simulink model "momentum_unload_test_super_simple"  (R2016b)
settings: Solver=VariableStepAuto  StartTime=0.0  StopTime=10  RelTol=1e-3
libraries: dynamics_lib x1, environment_lib x1, momentum_dump_lib x1, actuators_lib x1
settings Model: Creator=taylorreynolds  LastModifiedBy=evich

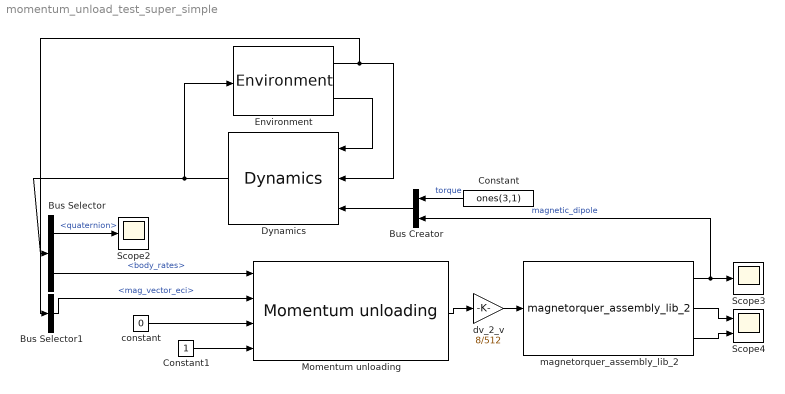
== system momentum_unload_test_super_simple ==
  Bus Creator : BusCreator  Inputs=2
  Bus Selector : BusSelector  OutputSignals=quaternion,body_rates
  Bus Selector1 : BusSelector  OutputSignals=mag_vector_eci
  Constant : Constant  Value=ones(3,1)
  Constant1 : Constant
  Dynamics : dynamics_lib/Dynamics
  Environment : environment_lib/Environment
  Momentum unloading : momentum_dump_lib/Momentum unloading
  Scope2 : Scope
  Scope3 : Scope
  Scope4 : Scope  NumInputPorts=2
  constant : Constant  Value=0
  dv_2_v : Gain  Gain=8/512
  magnetorquer_assembly_lib_2 : actuators_lib/Actuators/magnetorquer_assembly_lib_2
  wires:
  Environment/1 -> Bus Selector1/1, Dynamics/2
  Dynamics/1 -> Environment/1, Bus Selector/1
  Bus Selector/2 -> Momentum unloading/1  "<body_rates>"
  Bus Selector/1 -> Scope2/1  "<quaternion>"
  Bus Creator/1 -> Dynamics/3
  magnetorquer_assembly_lib_2/1 -> Scope3/1, Bus Creator/2  "magnetic_dipole"
  constant/1 -> Momentum unloading/3
  Momentum unloading/1 -> dv_2_v/1
  dv_2_v/1 -> magnetorquer_assembly_lib_2/1
  magnetorquer_assembly_lib_2/2 -> Scope4/1
  magnetorquer_assembly_lib_2/3 -> Scope4/2
  Constant1/1 -> Momentum unloading/4
  Bus Selector1/1 -> Momentum unloading/2  "<mag_vector_eci>"
  Constant/1 -> Bus Creator/1  "torque"
  Environment/2 -> Dynamics/1
